simulink model "prelab2sim"  (R2024a)
settings: Solver=ode45  StartTime=0.0  StopTime=3  MaxStep=0.001  RelTol=1e-3
settings Model: Creator=xinchen  LastModifiedBy=xinchen

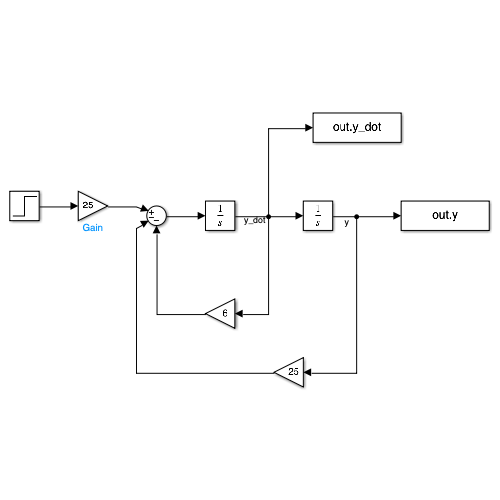
[thumbnail: Simulink's stored preview of the top-level diagram]
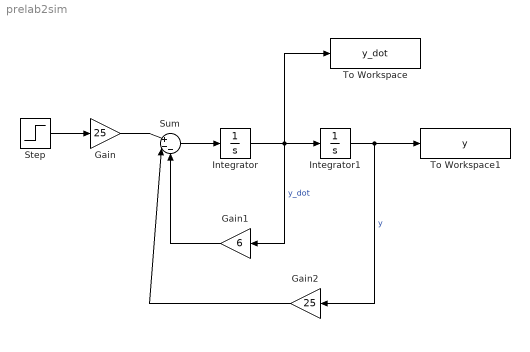
== system prelab2sim ==
  Gain : Gain  Gain=25
  Gain1 : Gain  Gain=6
  Gain2 : Gain  Gain=25
  Integrator : Integrator
  Integrator1 : Integrator
  Step : Step  Time=0  SampleTime=0
  Sum : Sum  Inputs=|+--
  To Workspace : ToWorkspace  VariableName=y_dot  SampleTime=-1
  To Workspace1 : ToWorkspace  VariableName=y  SampleTime=-1
  wires:
  Step/1 -> Gain/1
  Gain/1 -> Sum/1
  Integrator/1 -> To Workspace/1, Gain1/1, Integrator1/1  "y_dot"
  Sum/1 -> Integrator/1
  Integrator1/1 -> To Workspace1/1, Gain2/1  "y"
  Gain1/1 -> Sum/3
  Gain2/1 -> Sum/2
